simulink model "Verification_Tank1_Primitive"  (R2012b)
settings: Solver=FixedStepDiscrete  StartTime=0.0  StopTime=10.0  FixedStep=0.1  RelTol=1e-3
undefined symbols (not defined in the file): tank1_cross_section_area_m2, tank1_max_vol_m3, tank1_pump_flow_rate_m3s, tank1_valve_flow_rate_m3s
libraries: sldvlib x16
settings Model: Creator=Kerianne  LastModifiedBy=Kerianne
settings DataIOCC: SaveFormat=Structure
settings OptimizationCC: InlineParams=on

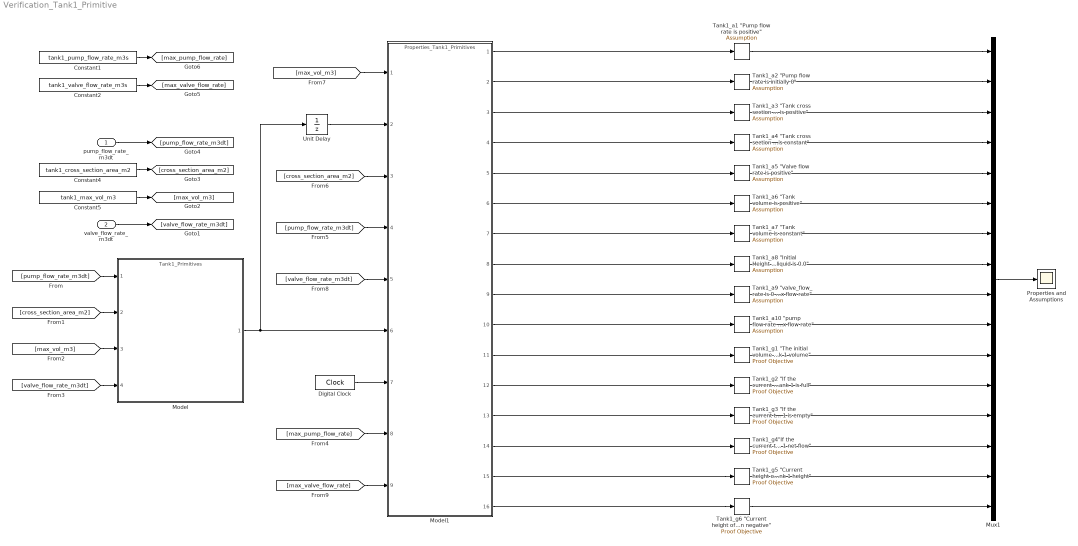
== system Verification_Tank1_Primitive ==
  pump_flow_rate_m3dt : Inport  OutDataTypeStr=double
  valve_flow_rate_m3dt : Inport  Port=2  OutDataTypeStr=double
  Constant1 : Constant  Value=tank1_pump_flow_rate_m3s
  Constant2 : Constant  Value=tank1_valve_flow_rate_m3s
  Constant4 : Constant  Value=tank1_cross_section_area_m2
  Constant5 : Constant  Value=tank1_max_vol_m3
  Digital Clock : DigitalClock  SampleTime=0.1
  Model : ModelReference  ModelNameDialog=Tank1_Primitives  SimulationMode=Normal  ModelReferenceVersion=1.30  CopyOfModelName=Tank1_Primitives  DefaultDataLogging=on
  Model1 : ModelReference  ModelNameDialog=Properties_Tank1_Primitives  SimulationMode=Normal  ModelReferenceVersion=1.39  CopyOfModelName=Properties_Tank1_Primitives  DefaultDataLogging=on
  Mux1 : Mux  Inputs=16
  Properties and Assumptions : Scope
      settings: ShowLegends=on
  "Tank1_a1 \"Pump flow rate is positive\"" : sldvlib/Objectives and Constraints/Assumption  enabled=on  customAVTBlockType=Assumption  intervals=true  initial=off  dispValues=on  outEnabled=on
      settings: AttributesFormatString=%<intervals>
  "Tank1_a10 \"pump flow rate is 0 or max flow rate\"" : sldvlib/Objectives and Constraints/Assumption  enabled=on  customAVTBlockType=Assumption  intervals=true  initial=off  dispValues=on  outEnabled=on
      settings: AttributesFormatString=%<intervals>
  "Tank1_a2 \"Pump flow rate is initially 0\"" : sldvlib/Objectives and Constraints/Assumption  enabled=on  customAVTBlockType=Assumption  intervals=true  initial=off  dispValues=on  outEnabled=on
      settings: AttributesFormatString=%<intervals>
  "Tank1_a3 \"Tank cross section area is positive\"" : sldvlib/Objectives and Constraints/Assumption  enabled=on  customAVTBlockType=Assumption  intervals=true  initial=off  dispValues=on  outEnabled=on
      settings: AttributesFormatString=%<intervals>
  "Tank1_a4 \"Tank cross section area is constant\"" : sldvlib/Objectives and Constraints/Assumption  enabled=on  customAVTBlockType=Assumption  intervals=true  initial=off  dispValues=on  outEnabled=on
      settings: AttributesFormatString=%<intervals>
  "Tank1_a5 \"Valve flow rate is positive\"" : sldvlib/Objectives and Constraints/Assumption  enabled=on  customAVTBlockType=Assumption  intervals=true  initial=off  dispValues=on  outEnabled=on
      settings: AttributesFormatString=%<intervals>
  "Tank1_a6 \"Tank volume is positive\"" : sldvlib/Objectives and Constraints/Assumption  enabled=on  customAVTBlockType=Assumption  intervals=true  initial=off  dispValues=on  outEnabled=on
      settings: AttributesFormatString=%<intervals>
  "Tank1_a7 \"Tank volume is constant\"" : sldvlib/Objectives and Constraints/Assumption  enabled=on  customAVTBlockType=Assumption  intervals=true  initial=off  dispValues=on  outEnabled=on
      settings: AttributesFormatString=%<intervals>
  "Tank1_a8 \"Initial Height of the liquid is 0.0\"" : sldvlib/Objectives and Constraints/Assumption  enabled=on  customAVTBlockType=Assumption  intervals=true  initial=off  dispValues=on  outEnabled=on
      settings: AttributesFormatString=%<intervals>
  "Tank1_a9 \"valve_flow_rate is 0 or max flow rate\"" : sldvlib/Objectives and Constraints/Assumption  enabled=on  customAVTBlockType=Assumption  intervals=true  initial=off  dispValues=on  outEnabled=on
      settings: AttributesFormatString=%<intervals>
  "Tank1_g1 \"The initial volume of tank 1 should be equivalent to the specified initial tank 1 volume\" " : sldvlib/Objectives and Constraints/Proof Objective  enabled=on  customAVTBlockType=Proof Objective  intervals=true  dispValues=on  outEnabled=on  enableStopSim=off
      settings: AttributesFormatString=%<intervals>
  "Tank1_g2 \"If the current tank 1 volume plus the tank 1 net flow is greater than the tank 1 maximum volume then tank 1 is full\"" : sldvlib/Objectives and Constraints/Proof Objective  enabled=on  customAVTBlockType=Proof Objective  intervals=true  dispValues=on  outEnabled=on  enableStopSim=off
      settings: AttributesFormatString=%<intervals>
  "Tank1_g3 \"If the current tank 1 volume plus the tank 1 net flow is less than the tank 1 minimum volume then tank 1 is empty\"" : sldvlib/Objectives and Constraints/Proof Objective  enabled=on  customAVTBlockType=Proof Objective  intervals=true  dispValues=on  outEnabled=on  enableStopSim=off
      settings: AttributesFormatString=%<intervals>
  "Tank1_g4\"If the current tank 1 volume plus the tank 1 net flow is greater than empty and less than the tank 1 maximum volume then the tank 1 volume changes by the tank 1 net flow\"" : sldvlib/Objectives and Constraints/Proof Objective  enabled=on  customAVTBlockType=Proof Objective  intervals=true  dispValues=on  outEnabled=on  enableStopSim=off
      settings: AttributesFormatString=%<intervals>
  "Tank1_g5 \"Current height of tank 1 is equal or less than the max tank 1 height\"" : sldvlib/Objectives and Constraints/Proof Objective  enabled=on  customAVTBlockType=Proof Objective  intervals=true  dispValues=on  outEnabled=on  enableStopSim=off
      settings: AttributesFormatString=%<intervals>
  "Tank1_g6 \"Current height of tank 1 is non negative\" " : sldvlib/Objectives and Constraints/Proof Objective  enabled=on  customAVTBlockType=Proof Objective  intervals=true  dispValues=on  outEnabled=on  enableStopSim=off
      settings: AttributesFormatString=%<intervals>
  Unit Delay : UnitDelay  SampleTime=-1
  wires:
  Model1/15 -> "Tank1_g5 \"Current height of tank 1 is equal or less than the max tank 1 height\""/1
  Model1/11 -> "Tank1_g1 \"The initial volume of tank 1 should be equivalent to the specified initial tank 1 volume\" "/1
  Model1/14 -> "Tank1_g4\"If the current tank 1 volume plus the tank 1 net flow is greater than empty and less than the tank 1 maximum volume then the tank 1 volume changes by the tank 1 net flow\""/1
  Model1/13 -> "Tank1_g3 \"If the current tank 1 volume plus the tank 1 net flow is less than the tank 1 minimum volume then tank 1 is empty\""/1
  Model1/12 -> "Tank1_g2 \"If the current tank 1 volume plus the tank 1 net flow is greater than the tank 1 maximum volume then tank 1 is full\""/1
  Model1/16 -> "Tank1_g6 \"Current height of tank 1 is non negative\" "/1
  Mux1/1 -> Properties and Assumptions/1
  Model/1 -> Unit Delay/1, Model1/6
  Digital Clock/1 -> Model1/7
  valve_flow_rate_m3dt/1 -> [valve_flow_rate_m3dt]
  pump_flow_rate_m3dt/1 -> [pump_flow_rate_m3dt]
  [valve_flow_rate_m3dt] -> Model1/5
  [pump_flow_rate_m3dt] -> Model1/4
  [cross_section_area_m2] -> Model1/3
  [max_vol_m3] -> Model1/1
  [valve_flow_rate_m3dt] -> Model/4
  [max_vol_m3] -> Model/3
  [cross_section_area_m2] -> Model/2
  [pump_flow_rate_m3dt] -> Model/1
  Model1/8 -> "Tank1_a8 \"Initial Height of the liquid is 0.0\""/1
  Model1/7 -> "Tank1_a7 \"Tank volume is constant\""/1
  Model1/6 -> "Tank1_a6 \"Tank volume is positive\""/1
  Model1/5 -> "Tank1_a5 \"Valve flow rate is positive\""/1
  Model1/4 -> "Tank1_a4 \"Tank cross section area is constant\""/1
  Model1/3 -> "Tank1_a3 \"Tank cross section area is positive\""/1
  Model1/2 -> "Tank1_a2 \"Pump flow rate is initially 0\""/1
  Model1/1 -> "Tank1_a1 \"Pump flow rate is positive\""/1
  "Tank1_a1 \"Pump flow rate is positive\""/1 -> Mux1/1
  "Tank1_a2 \"Pump flow rate is initially 0\""/1 -> Mux1/2
  "Tank1_a3 \"Tank cross section area is positive\""/1 -> Mux1/3
  "Tank1_a4 \"Tank cross section area is constant\""/1 -> Mux1/4
  "Tank1_a5 \"Valve flow rate is positive\""/1 -> Mux1/5
  "Tank1_a6 \"Tank volume is positive\""/1 -> Mux1/6
  "Tank1_a7 \"Tank volume is constant\""/1 -> Mux1/7
  "Tank1_a8 \"Initial Height of the liquid is 0.0\""/1 -> Mux1/8
  "Tank1_g1 \"The initial volume of tank 1 should be equivalent to the specified initial tank 1 volume\" "/1 -> Mux1/11
  "Tank1_g2 \"If the current tank 1 volume plus the tank 1 net flow is greater than the tank 1 maximum volume then tank 1 is full\""/1 -> Mux1/12
  "Tank1_g3 \"If the current tank 1 volume plus the tank 1 net flow is less than the tank 1 minimum volume then tank 1 is empty\""/1 -> Mux1/13
  "Tank1_g4\"If the current tank 1 volume plus the tank 1 net flow is greater than empty and less than the tank 1 maximum volume then the tank 1 volume changes by the tank 1 net flow\""/1 -> Mux1/14
  "Tank1_g5 \"Current height of tank 1 is equal or less than the max tank 1 height\""/1 -> Mux1/15
  "Tank1_g6 \"Current height of tank 1 is non negative\" "/1 -> Mux1/16
  Unit Delay/1 -> Model1/2
  Constant5/1 -> [max_vol_m3]
  Constant4/1 -> [cross_section_area_m2]
  Constant2/1 -> [max_valve_flow_rate]
  Constant1/1 -> [max_pump_flow_rate]
  [max_valve_flow_rate] -> Model1/9
  [max_pump_flow_rate] -> Model1/8
  Model1/9 -> "Tank1_a9 \"valve_flow_rate is 0 or max flow rate\""/1
  "Tank1_a9 \"valve_flow_rate is 0 or max flow rate\""/1 -> Mux1/9
  Model1/10 -> "Tank1_a10 \"pump flow rate is 0 or max flow rate\""/1
  "Tank1_a10 \"pump flow rate is 0 or max flow rate\""/1 -> Mux1/10
